simulink model "eCS_Algo_Simulation_2015b"  (R2015b)
settings: Solver=ode1  StartTime=0.0  StopTime=3  FixedStep=1/80000  RelTol=1e-3
PreLoadFcn:
  | if exist('tl_preloadfcn','file'), tl_preloadfcn(gcs,402); end
PostLoadFcn:
  | , if any(exist('dsrtsu_mdlpostloadfcn', 'file') == [2, 3, 6]), try dsrtsu_mdlpostloadfcn('Execute', bdroot); catch fprintf('Error in PostLoadFcn (dsrtsu_mdlpostloadfcn) for model "%s":\n %s\n', bdroot, lasterr); end, end,
  | if exist('tl_postloadfcn','file'), tl_postloadfcn(gcs,402); end
InitFcn:
  | Omegan=1.3024e+03;
  | xi=0.9; %0.48
  | K=0.1931;
  | K1=0.0198;
  | TauLocked=0.00255;
  | TauUnLocked=0.0042;
  | Kp=1/(2*K1);
  | Ki=Kp/((TauLocked+TauUnLocked)/2);
  | if exist('tlds_init','file'), tlds_init(gcs); end
StartFcn:
  | if exist('tlds_start','file'), tlds_start(gcs); end
StopFcn:
  | if exist('tlds_stop','file'), tlds_stop(gcs); end
model workspace (MAT data in the model file):
  au8PrevExecProfile = [0 0 0 0 0 0]
values from neighbouring files (symbols this model uses):
  AccSensor = 5    [Parameter_eCS_Algo.m]
  AlgoType = 0    [Parameter_eCS_Algo.m]
  Cxy = 1*0.017    (= 0.017)    [Acc_Init_SelV1.m]
  Cxz = 1*0.017    (= 0.017)    [Acc_Init_SelV1.m]
  Cyx = 1*0.017    (= 0.017)    [Acc_Init_SelV1.m]
  Cyz = 1*0.017    (= 0.017)    [Acc_Init_SelV1.m]
  Czx = 1*0.017    (= 0.017)    [Acc_Init_SelV1.m]
  Czy = 1*0.017    (= 0.017)    [Acc_Init_SelV1.m]
  Forced_Oscillation = 0    [Parameter_eCS_Algo.m]    (also in run_Rotation_sim.m = run)
  FreqTemperature = 10    [Acc_Init_SelV1.m]
  MaxSensorOffset = 0.3    [Acc_Init_SelV1.m]
  Mean_x_noise = 4e-3    (= 0.004)    [Acc_Init_SelV1.m]
  Mean_y_noise = 4e-3    (= 0.004)    [Acc_Init_SelV1.m]
  Mean_z_noise = 4e-3    (= 0.004)    [Acc_Init_SelV1.m]
  ODR = 8000    [Acc_Init_SelV1.m]
  offsetcorrection_on_off = 0    [Parameter_eCS_Algo.m]
  phi_pulse_rotation = 0    [Parameter_eCS_Algo.m]    (also in run_Rotation_sim.m = angle)
  pulsetype = 2    [Parameter_eCS_Algo.m]    (also in run_simulation.m = j; run_simulation_ActiveX.m = j)
  Range = 4    [Acc_Init_SelV1.m]
  sensitivity_optimisation = 0    [Parameter_eCS_Algo.m]
  TempBias = 0    [Acc_Init_SelV1.m]
  TemperatureAmp = 0    [Acc_Init_SelV1.m]
  Var_x_noise = 1.84e-9    (= 1.84e-09)    [Acc_Init_SelV1.m]
  Var_y_noise = 2.025e-09    [Acc_Init_SelV1.m]
  Var_z_noise = 1.374e-09    [Acc_Init_SelV1.m]
  w_x = 2*pi*F_x    (= 376.991118431)    [Acc_Init_SelV1.m]
  w_y = 2*pi*F_y    (= 376.991118431)    [Acc_Init_SelV1.m]
  w_z = 2*pi*F_z    (= 376.991118431)    [Acc_Init_SelV1.m]
  x_max_temp_drift = 0.061    [Acc_Init_SelV1.m]
  x_offset_enable = 0    [Acc_Init_SelV1.m]
  x_run_to_run_drift = 0.0    (= 0)    [Acc_Init_SelV1.m]
  x_temp_co_drift = 0.000    (= 0)    [Acc_Init_SelV1.m]
  Xi_x = 0.7    [Acc_Init_SelV1.m]
  Xi_y = 0.7    [Acc_Init_SelV1.m]
  Xi_z = 0.7    [Acc_Init_SelV1.m]
  y_max_temp_drift = 0.061    [Acc_Init_SelV1.m]
  y_offset_enable = 0    [Acc_Init_SelV1.m]
  y_run_to_run_drift = 0.0    (= 0)    [Acc_Init_SelV1.m]
  y_temp_co_drift = 0.000    (= 0)    [Acc_Init_SelV1.m]
  z_max_temp_drift = 0.13    [Acc_Init_SelV1.m]
  z_offset_enable = 0    [Acc_Init_SelV1.m]
  z_run_to_run_drift = 0.0    (= 0)    [Acc_Init_SelV1.m]
  z_temp_co_drift = 0.000    (= 0)    [Acc_Init_SelV1.m]
undefined symbols (not defined in the file or in its folder): controller_sample_rate, ddv, DiscIntNeverNeededParam, gmw_roada_x__m_s__, gmw_roada_y__m_s__, gmw_roadtime_2kHz, KSF_50_a_x, KSF_50_a_y, KSF_50_time, KSG_30_a_x, KSG_30_a_y, KSG_30_time, Meldorf_HindenburgstraAcceleration_x__m_s_2_, Meldorf_HindenburgstraAcceleration_y__m_s_2_, Meldorf_HindenburgstraAcceleration_z__m_s_2_, Meldorf_HindenburgstraTime__s_, pulse_FF27, pulse_MPDB, pulse_ODB40, pulse_ODB64, pulse_USNCAP, pulsetime_FF27, pulsetime_MPDB, pulsetime_ODB40, pulsetime_ODB64, pulsetime_USNCAP, Rauasphalt_60_a_x, Rauasphalt_60_a_y, Rauasphalt_60_time, sigbuilder_block, VW_416_2kHza_x_2kHz, VW_416_2kHza_y_2kHz, VW_416_2kHztime_2kHz
libraries: simulink x29, tllib x23, tl_autosar_lib x15, simulink_extras x7, LIB_TF_G_111 x2, LIB_TF_G_12_StepControl x2, LIB_TF_G_112 x1, dspsigops x1
(part 4 of 13)

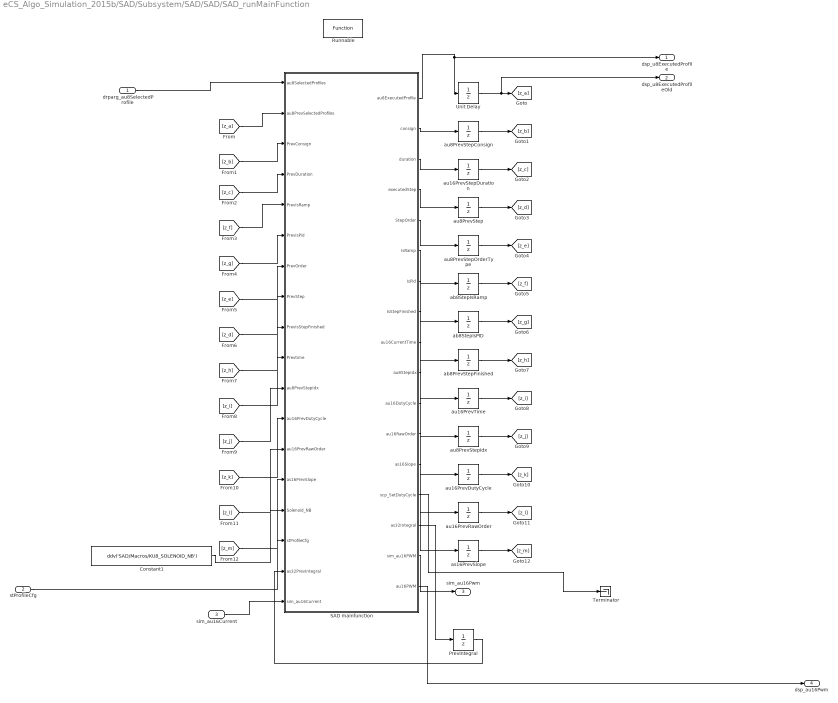
== system eCS_Algo_Simulation_2015b/SAD/Subsystem/SAD/SAD/SAD_runMainFunction ==
  drparg_au8SelectedProfile : Inport  PortDimensions=6  mask(TL_Inport){data={'logdata',{'loggingmode',1},'autosar',{'useautosarcommunication',1,'senderreceiverport','prrFsmProfile','dataelement','au8SelectedProfile'},'date',738567.35573128471}}
      settings: CopyFcn=if exist('tl_reset_reviewflag') == 2, tl_reset_reviewflag(gcbh); end  DeleteFcn=if exist('delete_tlblock','file')==2,delete_tlblock(gcbh);end  NameChangeFcn=if exist('rename_tlblock','file')==2,rename_tlblock(gcbh);end  OpenFcn=if exist('tl_open_blockdlg','file')==2,tl_open_blockdlg(gcbh);else,open_system(gcbh,'parameter');end
      mask Help: eval(['if exist(''tl_online_help'',''file'') == 2, tl_online_help(''Topic'',''TL_Inport''),else, web([''jar:file:///'',matlabroot,''/help/toolbox/simulink/help.jar!/slref/' lower(get_param(gcbh,'Blocktype')) '.html''], ''-helpbrowser''),end'])
      mask Display: plot([0.2 0.35 NaN 0.65 0.8],[0 1 NaN 0 1]);
  stProfileCfg : Inport  Port=2  mask(TL_BusInport){data={'#autoscaling',2,'#message',2,'#output',2,'#logdata',2,'logdata#1',{'loggingmode',1},'logdata#2',{'loggingmode',1},'signals',{{'stProfileCfg',{'au8FollowingProfile';'au8LastStep'}}},'autosar',{'useautosarcommunication',1,'kind',3,'interrunnablevariable','stProfileCfg'},'date',738430.41690388892}}
      settings: CopyFcn=if exist('tl_reset_reviewflag') == 2, tl_reset_reviewflag(gcbh); end  DeleteFcn=if exist('delete_tlblock','file')==2,delete_tlblock(gcbh);end  NameChangeFcn=if exist('rename_tlblock','file')==2,rename_tlblock(gcbh);end  OpenFcn=if exist('tl_open_blockdlg','file')==2,tl_open_blockdlg(gcbh);else,open_system(gcbh,'parameter');end
      mask Help: eval(['if exist(''tl_online_help'',''file'') == 2, tl_online_help(''Topic'',''TL_Inport''),else, web([''jar:file:///'',matlabroot,''/help/toolbox/simulink/help.jar!/slref/' lower(get_param(gcbh,'Blocktype')) '.html''], ''-helpbrowser''),end'])
      mask Display: plot([0.2 0.35 NaN 0.65 0.8],[0 1 NaN 0 1]);
  sim_au16Current : Inport  Port=3
  Constant1 : Constant  Value=ddv('SAD/Macros/KU8_SOLENOID_NB')  mask(TL_Constant){data={'output',{'variable','SAD/Macros/KU8_SOLENOID_NB'},'date',738430.41690414352}}
      settings: CopyFcn=if exist('tl_reset_reviewflag') == 2, tl_reset_reviewflag(gcbh); end  DeleteFcn=if exist('delete_tlblock','file')==2,delete_tlblock(gcbh);end  NameChangeFcn=if exist('rename_tlblock','file')==2,rename_tlblock(gcbh);end  OpenFcn=if exist('tl_open_blockdlg','file')==2,tl_open_blockdlg(gcbh);else,open_system(gcbh,'parameter');end
      mask Help: eval(['if exist(''tl_online_help'',''file'') == 2, tl_online_help(''Topic'',''TL_Constant''),else, web([''jar:file:///'',matlabroot,''/help/toolbox/simulink/help.jar!/slref/' lower(get_param(gcbh,'Blocktype')) '.html''], ''-helpbrowser''),end'])
      mask Display: plot([-0.1, 1.05, NaN, -0.1, 1.05],[.01, .01, NaN, .99, .99]);
  PrevIntegral : UnitDelay  InitialCondition=ddv('SAD/Vars/Steps/as32PrevIntegral')  SampleTime=-1  mask(TL_UnitDelay){data={'logdata',{'loggingmode',1},'output',{'type','Int32','scaling','scPID'},'state',{'variable','SAD/Vars/Steps/as32PrevIntegral'},'date',738433.59244626155}}
      settings: CopyFcn=if exist('tl_reset_reviewflag') == 2, tl_reset_reviewflag(gcbh); end  DeleteFcn=if exist('delete_tlblock','file')==2,delete_tlblock(gcbh);end  NameChangeFcn=if exist('rename_tlblock','file')==2,rename_tlblock(gcbh);end  OpenFcn=if exist('tl_open_blockdlg','file')==2,tl_open_blockdlg(gcbh);else,open_system(gcbh,'parameter');end
      mask Help: eval(['if exist(''tl_online_help'',''file'') == 2, tl_online_help(''Topic'',''TL_UnitDelay''),else, web([''jar:file:///'',matlabroot,''/help/toolbox/simulink/help.jar!/slref/' lower(get_param(gcbh,'Blocktype')) '.html''], ''-helpbrowser''),end'])
      mask Display: plot([-0.1, 1.05, NaN, -0.1, 1.05],[.01, .01, NaN, .99, .99]);
  Runnable : tllib/Function  data={'autosar',{'useautosarspecification',1,'softwarecomponent','AUTOLIV/SoftwareComponents/SAD/SAD','runnable','SAD_runMainFunction'},'date',738433.36681372684}  displayString=RUNNABLE
  SAD mainfunction : Subsystem  TreatAsAtomicUnit=on
  Terminator : Terminator
  Unit Delay : UnitDelay  InitialCondition=ddv('SAD/Vars/Profiles/au8PrevExecProfile')  SampleTime=-1  mask(TL_UnitDelay){data={'output',{'inheritscaling',1},'state',{'variable','SAD/Vars/Profiles/au8PrevExecProfile'},'date',738430.41691655095}}
      settings: CopyFcn=if exist('tl_reset_reviewflag') == 2, tl_reset_reviewflag(gcbh); end  DeleteFcn=if exist('delete_tlblock','file')==2,delete_tlblock(gcbh);end  NameChangeFcn=if exist('rename_tlblock','file')==2,rename_tlblock(gcbh);end  OpenFcn=if exist('tl_open_blockdlg','file')==2,tl_open_blockdlg(gcbh);else,open_system(gcbh,'parameter');end
      mask Help: eval(['if exist(''tl_online_help'',''file'') == 2, tl_online_help(''Topic'',''TL_UnitDelay''),else, web([''jar:file:///'',matlabroot,''/help/toolbox/simulink/help.jar!/slref/' lower(get_param(gcbh,'Blocktype')) '.html''], ''-helpbrowser''),end'])
      mask Display: plot([-0.1, 1.05, NaN, -0.1, 1.05],[.01, .01, NaN, .99, .99]);
  ab8PrevStepFinished : UnitDelay  InitialCondition=ddv('SAD/Vars/Steps/ab8PrevIsStepFinished')  SampleTime=-1  mask(TL_UnitDelay){data={'logdata',{'loggingmode',1},'output',{'type','Bool'},'state',{'variable','SAD/Vars/Steps/ab8PrevIsStepFinished'},'date',738430.41691681708}}
      settings: CopyFcn=if exist('tl_reset_reviewflag') == 2, tl_reset_reviewflag(gcbh); end  DeleteFcn=if exist('delete_tlblock','file')==2,delete_tlblock(gcbh);end  NameChangeFcn=if exist('rename_tlblock','file')==2,rename_tlblock(gcbh);end  OpenFcn=if exist('tl_open_blockdlg','file')==2,tl_open_blockdlg(gcbh);else,open_system(gcbh,'parameter');end
      mask Help: eval(['if exist(''tl_online_help'',''file'') == 2, tl_online_help(''Topic'',''TL_UnitDelay''),else, web([''jar:file:///'',matlabroot,''/help/toolbox/simulink/help.jar!/slref/' lower(get_param(gcbh,'Blocktype')) '.html''], ''-helpbrowser''),end'])
      mask Display: plot([-0.1, 1.05, NaN, -0.1, 1.05],[.01, .01, NaN, .99, .99]);
  ab8StepIsPID : UnitDelay  InitialCondition=ddv('SAD/Vars/Steps/astPrevSteps/Components/ab8IsPID')  SampleTime=-1  mask(TL_UnitDelay){data={'output',{'inheritscaling',1},'state',{'variable','SAD/Vars/Steps/astPrevSteps/Components/ab8IsPID'},'date',738430.41691716434}}
      settings: CopyFcn=if exist('tl_reset_reviewflag') == 2, tl_reset_reviewflag(gcbh); end  DeleteFcn=if exist('delete_tlblock','file')==2,delete_tlblock(gcbh);end  NameChangeFcn=if exist('rename_tlblock','file')==2,rename_tlblock(gcbh);end  OpenFcn=if exist('tl_open_blockdlg','file')==2,tl_open_blockdlg(gcbh);else,open_system(gcbh,'parameter');end
      mask Help: eval(['if exist(''tl_online_help'',''file'') == 2, tl_online_help(''Topic'',''TL_UnitDelay''),else, web([''jar:file:///'',matlabroot,''/help/toolbox/simulink/help.jar!/slref/' lower(get_param(gcbh,'Blocktype')) '.html''], ''-helpbrowser''),end'])
      mask Display: plot([-0.1, 1.05, NaN, -0.1, 1.05],[.01, .01, NaN, .99, .99]);
  ab8StepIsRamp : UnitDelay  InitialCondition=ddv('SAD/Vars/Steps/astPrevSteps/Components/ab8IsRamp')  SampleTime=-1  mask(TL_UnitDelay){data={'logdata',{'loggingmode',1},'output',{'inheritscaling',1},'state',{'variable','SAD/Vars/Steps/astPrevSteps/Components/ab8IsRamp'},'date',738430.41691743059}}
      settings: CopyFcn=if exist('tl_reset_reviewflag') == 2, tl_reset_reviewflag(gcbh); end  DeleteFcn=if exist('delete_tlblock','file')==2,delete_tlblock(gcbh);end  NameChangeFcn=if exist('rename_tlblock','file')==2,rename_tlblock(gcbh);end  OpenFcn=if exist('tl_open_blockdlg','file')==2,tl_open_blockdlg(gcbh);else,open_system(gcbh,'parameter');end
      mask Help: eval(['if exist(''tl_online_help'',''file'') == 2, tl_online_help(''Topic'',''TL_UnitDelay''),else, web([''jar:file:///'',matlabroot,''/help/toolbox/simulink/help.jar!/slref/' lower(get_param(gcbh,'Blocktype')) '.html''], ''-helpbrowser''),end'])
      mask Display: plot([-0.1, 1.05, NaN, -0.1, 1.05],[.01, .01, NaN, .99, .99]);
  as16PrevSlope : UnitDelay  InitialCondition=ddv('SAD/Vars/Steps/as16PrevSlope')  SampleTime=-1  mask(TL_UnitDelay){data={'output',{'inheritscaling',1},'state',{'variable','SAD/Vars/Steps/as16PrevSlope'},'date',738430.41691781254}}
      settings: CopyFcn=if exist('tl_reset_reviewflag') == 2, tl_reset_reviewflag(gcbh); end  DeleteFcn=if exist('delete_tlblock','file')==2,delete_tlblock(gcbh);end  NameChangeFcn=if exist('rename_tlblock','file')==2,rename_tlblock(gcbh);end  OpenFcn=if exist('tl_open_blockdlg','file')==2,tl_open_blockdlg(gcbh);else,open_system(gcbh,'parameter');end
      mask Help: eval(['if exist(''tl_online_help'',''file'') == 2, tl_online_help(''Topic'',''TL_UnitDelay''),else, web([''jar:file:///'',matlabroot,''/help/toolbox/simulink/help.jar!/slref/' lower(get_param(gcbh,'Blocktype')) '.html''], ''-helpbrowser''),end'])
      mask Display: plot([-0.1, 1.05, NaN, -0.1, 1.05],[.01, .01, NaN, .99, .99]);
  au16PrevDutyCycle : UnitDelay  InitialCondition=ddv('SAD/Vars/Steps/au16PrevDutyCycle')  SampleTime=-1  mask(TL_UnitDelay){data={'output',{'type','UInt16'},'state',{'variable','SAD/Vars/Steps/au16PrevDutyCycle'},'date',738566.69629486115}}
      settings: CopyFcn=if exist('tl_reset_reviewflag') == 2, tl_reset_reviewflag(gcbh); end  DeleteFcn=if exist('delete_tlblock','file')==2,delete_tlblock(gcbh);end  NameChangeFcn=if exist('rename_tlblock','file')==2,rename_tlblock(gcbh);end  OpenFcn=if exist('tl_open_blockdlg','file')==2,tl_open_blockdlg(gcbh);else,open_system(gcbh,'parameter');end
      mask Help: eval(['if exist(''tl_online_help'',''file'') == 2, tl_online_help(''Topic'',''TL_UnitDelay''),else, web([''jar:file:///'',matlabroot,''/help/toolbox/simulink/help.jar!/slref/' lower(get_param(gcbh,'Blocktype')) '.html''], ''-helpbrowser''),end'])
      mask Display: plot([-0.1, 1.05, NaN, -0.1, 1.05],[.01, .01, NaN, .99, .99]);
  au16PrevRawOrder : UnitDelay  InitialCondition=ddv('SAD/Vars/Steps/au16PrevRawOrder')  SampleTime=-1  mask(TL_UnitDelay){data={'output',{'inheritscaling',1},'state',{'variable','SAD/Vars/Steps/au16PrevRawOrder'},'date',738430.41691839125}}
      settings: CopyFcn=if exist('tl_reset_reviewflag') == 2, tl_reset_reviewflag(gcbh); end  DeleteFcn=if exist('delete_tlblock','file')==2,delete_tlblock(gcbh);end  NameChangeFcn=if exist('rename_tlblock','file')==2,rename_tlblock(gcbh);end  OpenFcn=if exist('tl_open_blockdlg','file')==2,tl_open_blockdlg(gcbh);else,open_system(gcbh,'parameter');end
      mask Help: eval(['if exist(''tl_online_help'',''file'') == 2, tl_online_help(''Topic'',''TL_UnitDelay''),else, web([''jar:file:///'',matlabroot,''/help/toolbox/simulink/help.jar!/slref/' lower(get_param(gcbh,'Blocktype')) '.html''], ''-helpbrowser''),end'])
      mask Display: plot([-0.1, 1.05, NaN, -0.1, 1.05],[.01, .01, NaN, .99, .99]);
  au16PrevStepDuration : UnitDelay  InitialCondition=ddv('SAD/Vars/Steps/astPrevSteps/Components/au16Duration')  SampleTime=-1  mask(TL_UnitDelay){data={'logdata',{'loggingmode',1},'output',{'inheritscaling',1},'state',{'variable','SAD/Vars/Steps/astPrevSteps/Components/au16Duration'},'date',738430.41691861115}}
      settings: CopyFcn=if exist('tl_reset_reviewflag') == 2, tl_reset_reviewflag(gcbh); end  DeleteFcn=if exist('delete_tlblock','file')==2,delete_tlblock(gcbh);end  NameChangeFcn=if exist('rename_tlblock','file')==2,rename_tlblock(gcbh);end  OpenFcn=if exist('tl_open_blockdlg','file')==2,tl_open_blockdlg(gcbh);else,open_system(gcbh,'parameter');end
      mask Help: eval(['if exist(''tl_online_help'',''file'') == 2, tl_online_help(''Topic'',''TL_UnitDelay''),else, web([''jar:file:///'',matlabroot,''/help/toolbox/simulink/help.jar!/slref/' lower(get_param(gcbh,'Blocktype')) '.html''], ''-helpbrowser''),end'])
      mask Display: plot([-0.1, 1.05, NaN, -0.1, 1.05],[.01, .01, NaN, .99, .99]);
  au16PrevTime : UnitDelay  InitialCondition=ddv('SAD/Vars/Steps/au16PrevTime')  SampleTime=-1  mask(TL_UnitDelay){data={'logdata',{'loggingmode',1},'output',{'inheritscaling',1},'state',{'variable','SAD/Vars/Steps/au16PrevTime'},'date',738430.41691896995}}
      settings: CopyFcn=if exist('tl_reset_reviewflag') == 2, tl_reset_reviewflag(gcbh); end  DeleteFcn=if exist('delete_tlblock','file')==2,delete_tlblock(gcbh);end  NameChangeFcn=if exist('rename_tlblock','file')==2,rename_tlblock(gcbh);end  OpenFcn=if exist('tl_open_blockdlg','file')==2,tl_open_blockdlg(gcbh);else,open_system(gcbh,'parameter');end
      mask Help: eval(['if exist(''tl_online_help'',''file'') == 2, tl_online_help(''Topic'',''TL_UnitDelay''),else, web([''jar:file:///'',matlabroot,''/help/toolbox/simulink/help.jar!/slref/' lower(get_param(gcbh,'Blocktype')) '.html''], ''-helpbrowser''),end'])
      mask Display: plot([-0.1, 1.05, NaN, -0.1, 1.05],[.01, .01, NaN, .99, .99]);
  au8PrevStep : UnitDelay  InitialCondition=ddv('SAD/Vars/Steps/au8PrevExecStep')  SampleTime=-1  mask(TL_UnitDelay){data={'output',{'inheritscaling',1},'state',{'variable','SAD/Vars/Steps/au8PrevExecStep'},'date',738430.41691923607}}
      settings: CopyFcn=if exist('tl_reset_reviewflag') == 2, tl_reset_reviewflag(gcbh); end  DeleteFcn=if exist('delete_tlblock','file')==2,delete_tlblock(gcbh);end  NameChangeFcn=if exist('rename_tlblock','file')==2,rename_tlblock(gcbh);end  OpenFcn=if exist('tl_open_blockdlg','file')==2,tl_open_blockdlg(gcbh);else,open_system(gcbh,'parameter');end
      mask Help: eval(['if exist(''tl_online_help'',''file'') == 2, tl_online_help(''Topic'',''TL_UnitDelay''),else, web([''jar:file:///'',matlabroot,''/help/toolbox/simulink/help.jar!/slref/' lower(get_param(gcbh,'Blocktype')) '.html''], ''-helpbrowser''),end'])
      mask Display: plot([-0.1, 1.05, NaN, -0.1, 1.05],[.01, .01, NaN, .99, .99]);
  au8PrevStepConsign : UnitDelay  InitialCondition=ddv('SAD/Vars/Steps/astPrevSteps/Components/au8Consign')  SampleTime=-1  mask(TL_UnitDelay){data={'output',{'inheritscaling',1},'state',{'variable','SAD/Vars/Steps/astPrevSteps/Components/au8Consign'},'date',738430.41691947915}}
      settings: CopyFcn=if exist('tl_reset_reviewflag') == 2, tl_reset_reviewflag(gcbh); end  DeleteFcn=if exist('delete_tlblock','file')==2,delete_tlblock(gcbh);end  NameChangeFcn=if exist('rename_tlblock','file')==2,rename_tlblock(gcbh);end  OpenFcn=if exist('tl_open_blockdlg','file')==2,tl_open_blockdlg(gcbh);else,open_system(gcbh,'parameter');end
      mask Help: eval(['if exist(''tl_online_help'',''file'') == 2, tl_online_help(''Topic'',''TL_UnitDelay''),else, web([''jar:file:///'',matlabroot,''/help/toolbox/simulink/help.jar!/slref/' lower(get_param(gcbh,'Blocktype')) '.html''], ''-helpbrowser''),end'])
      mask Display: plot([-0.1, 1.05, NaN, -0.1, 1.05],[.01, .01, NaN, .99, .99]);
  au8PrevStepIdx : UnitDelay  InitialCondition=ddv('SAD/Vars/Steps/au8PrevStepIdx')  SampleTime=-1  mask(TL_UnitDelay){data={'logdata',{'loggingmode',1},'output',{'inheritscaling',1},'state',{'variable','SAD/Vars/Steps/au8PrevStepIdx'},'date',738430.41691981477}}
      settings: CopyFcn=if exist('tl_reset_reviewflag') == 2, tl_reset_reviewflag(gcbh); end  DeleteFcn=if exist('delete_tlblock','file')==2,delete_tlblock(gcbh);end  NameChangeFcn=if exist('rename_tlblock','file')==2,rename_tlblock(gcbh);end  OpenFcn=if exist('tl_open_blockdlg','file')==2,tl_open_blockdlg(gcbh);else,open_system(gcbh,'parameter');end
      mask Help: eval(['if exist(''tl_online_help'',''file'') == 2, tl_online_help(''Topic'',''TL_UnitDelay''),else, web([''jar:file:///'',matlabroot,''/help/toolbox/simulink/help.jar!/slref/' lower(get_param(gcbh,'Blocktype')) '.html''], ''-helpbrowser''),end'])
      mask Display: plot([-0.1, 1.05, NaN, -0.1, 1.05],[.01, .01, NaN, .99, .99]);
  au8PrevStepOrderType : UnitDelay  InitialCondition=ddv('SAD/Vars/Steps/astPrevSteps/Components/au8OrderType')  SampleTime=-1  mask(TL_UnitDelay){data={'output',{'inheritscaling',1},'state',{'variable','SAD/Vars/Steps/astPrevSteps/Components/au8OrderType'},'date',738430.41692012735}}
      settings: CopyFcn=if exist('tl_reset_reviewflag') == 2, tl_reset_reviewflag(gcbh); end  DeleteFcn=if exist('delete_tlblock','file')==2,delete_tlblock(gcbh);end  NameChangeFcn=if exist('rename_tlblock','file')==2,rename_tlblock(gcbh);end  OpenFcn=if exist('tl_open_blockdlg','file')==2,tl_open_blockdlg(gcbh);else,open_system(gcbh,'parameter');end
      mask Help: eval(['if exist(''tl_online_help'',''file'') == 2, tl_online_help(''Topic'',''TL_UnitDelay''),else, web([''jar:file:///'',matlabroot,''/help/toolbox/simulink/help.jar!/slref/' lower(get_param(gcbh,'Blocktype')) '.html''], ''-helpbrowser''),end'])
      mask Display: plot([-0.1, 1.05, NaN, -0.1, 1.05],[.01, .01, NaN, .99, .99]);
  dsp_u8ExecutedProfile : Outport  PortDimensions=6  mask(TL_Outport){data={'logdata',{'loggingmode',1},'autosar',{'useautosarcommunication',1,'senderreceiverport','psrExecutedProfiles','dataelement','u8ExecutedProfile'},'date',738430.41692024306}}
      settings: CopyFcn=if exist('tl_reset_reviewflag') == 2, tl_reset_reviewflag(gcbh); end  DeleteFcn=if exist('delete_tlblock','file')==2,delete_tlblock(gcbh);end  NameChangeFcn=if exist('rename_tlblock','file')==2,rename_tlblock(gcbh);end  OpenFcn=if exist('tl_open_blockdlg','file')==2,tl_open_blockdlg(gcbh);else,open_system(gcbh,'parameter');end
      mask Help: eval(['if exist(''tl_online_help'',''file'') == 2, tl_online_help(''Topic'',''TL_Outport''),else, web([''jar:file:///'',matlabroot,''/help/toolbox/simulink/help.jar!/slref/' lower(get_param(gcbh,'Blocktype')) '.html''], ''-helpbrowser''),end'])
      mask Display: plot([0.2 0.35 NaN 0.65 0.8],[0 1 NaN 0 1]);
  dsp_u8ExecutedProfileOld : Outport  Port=2  PortDimensions=6  mask(TL_Outport){data={'autosar',{'useautosarcommunication',1,'senderreceiverport','psrExecutedProfiles','dataelement','u8ExecutedProfileOld'},'date',738430.4169204745}}
      settings: CopyFcn=if exist('tl_reset_reviewflag') == 2, tl_reset_reviewflag(gcbh); end  DeleteFcn=if exist('delete_tlblock','file')==2,delete_tlblock(gcbh);end  NameChangeFcn=if exist('rename_tlblock','file')==2,rename_tlblock(gcbh);end  OpenFcn=if exist('tl_open_blockdlg','file')==2,tl_open_blockdlg(gcbh);else,open_system(gcbh,'parameter');end
      mask Help: eval(['if exist(''tl_online_help'',''file'') == 2, tl_online_help(''Topic'',''TL_Outport''),else, web([''jar:file:///'',matlabroot,''/help/toolbox/simulink/help.jar!/slref/' lower(get_param(gcbh,'Blocktype')) '.html''], ''-helpbrowser''),end'])
      mask Display: plot([0.2 0.35 NaN 0.65 0.8],[0 1 NaN 0 1]);
  sim_au16Pwm : Outport  Port=3
  dsp_au16Pwm : Outport  Port=4  PortDimensions=6  mask(TL_Outport){data={'logdata',{'loggingmode',1},'autosar',{'useautosarcommunication',1,'senderreceiverport','pseSolenoidPWM','dataelement','au16Pwm'},'date',738496.37130460644}}
      settings: CopyFcn=if exist('tl_reset_reviewflag') == 2, tl_reset_reviewflag(gcbh); end  DeleteFcn=if exist('delete_tlblock','file')==2,delete_tlblock(gcbh);end  NameChangeFcn=if exist('rename_tlblock','file')==2,rename_tlblock(gcbh);end  OpenFcn=if exist('tl_open_blockdlg','file')==2,tl_open_blockdlg(gcbh);else,open_system(gcbh,'parameter');end
      mask Help: eval(['if exist(''tl_online_help'',''file'') == 2, tl_online_help(''Topic'',''TL_Outport''),else, web([''jar:file:///'',matlabroot,''/help/toolbox/simulink/help.jar!/slref/' lower(get_param(gcbh,'Blocktype')) '.html''], ''-helpbrowser''),end'])
      mask Display: plot([0.2 0.35 NaN 0.65 0.8],[0 1 NaN 0 1]);
  wires:
  SAD mainfunction/1(au8ExecutedProfile) -> Unit Delay/1, dsp_u8ExecutedProfile/1
  Unit Delay/1 -> dsp_u8ExecutedProfileOld/1, [z_a]
  drparg_au8SelectedProfile/1 -> SAD mainfunction/1(au8SelectedProfiles)
  SAD mainfunction/2(consign) -> au8PrevStepConsign/1
  SAD mainfunction/3(duration) -> au16PrevStepDuration/1
  SAD mainfunction/8(IsStepFinished) -> ab8PrevStepFinished/1
  SAD mainfunction/7(IsPid) -> ab8StepIsPID/1
  SAD mainfunction/6(IsRamp) -> ab8StepIsRamp/1
  SAD mainfunction/5(StepOrder) -> au8PrevStepOrderType/1
  SAD mainfunction/4(executedStep) -> au8PrevStep/1
  [z_a] -> SAD mainfunction/2(au8PrevSelectedProfiles)
  au8PrevStepConsign/1 -> [z_b]
  au16PrevStepDuration/1 -> [z_c]
  au8PrevStep/1 -> [z_d]
  au8PrevStepOrderType/1 -> [z_e]
  ab8StepIsRamp/1 -> [z_f]
  ab8StepIsPID/1 -> [z_g]
  ab8PrevStepFinished/1 -> [z_h]
  [z_b] -> SAD mainfunction/3(PrevConsign)
  [z_c] -> SAD mainfunction/4(PrevDuration)
  [z_f] -> SAD mainfunction/5(PrevIsRamp)
  [z_g] -> SAD mainfunction/6(PrevIsPid)
  [z_e] -> SAD mainfunction/7(PrevOrder)
  [z_d] -> SAD mainfunction/8(PrevStep)
  [z_h] -> SAD mainfunction/9(PrevIsStepFinished)
  au16PrevTime/1 -> [z_i]
  SAD mainfunction/9(au16CurrentTime) -> au16PrevTime/1
  [z_i] -> SAD mainfunction/10(Prevtime)
  SAD mainfunction/10(au8StepIdx) -> au8PrevStepIdx/1
  au8PrevStepIdx/1 -> [z_j]
  [z_j] -> SAD mainfunction/11(au8PrevStepIdx)
  [z_k] -> SAD mainfunction/12(au16PrevDutyCycle)
  SAD mainfunction/11(au16DutyCycle) -> au16PrevDutyCycle/1
  au16PrevDutyCycle/1 -> [z_k]
  SAD mainfunction/12(au16RawOrder) -> au16PrevRawOrder/1
  SAD mainfunction/13(as16Slope) -> as16PrevSlope/1
  au16PrevRawOrder/1 -> [z_l]
  as16PrevSlope/1 -> [z_m]
  [z_l] -> SAD mainfunction/13(au16PrevRawOrder)
  [z_m] -> SAD mainfunction/14(as16PrevSlope)
  Constant1/1 -> SAD mainfunction/15(Solenoid_NB)
  stProfileCfg/1 -> SAD mainfunction/16(stProfileCfg)
  SAD mainfunction/14(scp_SetDutyCycle) -> Terminator/1
  SAD mainfunction/15(as32Integral) -> PrevIntegral/1
  PrevIntegral/1 -> SAD mainfunction/17(as32PrevIntegral)
  SAD mainfunction/16(sim_au16PWM) -> sim_au16Pwm/1
  sim_au16Current/1 -> SAD mainfunction/18(sim_au16Current)
  SAD mainfunction/17(au16PWM) -> dsp_au16Pwm/1

== system eCS_Algo_Simulation_2015b/eCS/Subsystem/eCS/eCS/eCS_runMainFunction ==
  drparg_stAccelMtrPerSecSqd : Inport  mask(TL_BusInport){data={'#autoscaling',3,'#message',3,'#output',3,'#logdata',3,'logdata#1',{'loggingmode',1},'logdata#2',{'loggingmode',1},'logdata#3',{'loggingmode',1},'signals',{{'stAccelMtrPerSecSqd',{'s16Ax';'s16Ay';'s16Az'}}},'autosar',{'useautosarcommunication',1,'senderreceiverport','prrAccelMtrPerSecSqd','dataelement','stAccelMtrPerSecSqd'},'date',738573.7191865046}}
      settings: CopyFcn=if exist('tl_reset_reviewflag') == 2, tl_reset_reviewflag(gcbh); end  DeleteFcn=if exist('delete_tlblock','file')==2,delete_tlblock(gcbh);end  NameChangeFcn=if exist('rename_tlblock','file')==2,rename_tlblock(gcbh);end  OpenFcn=if exist('tl_open_blockdlg','file')==2,tl_open_blockdlg(gcbh);else,open_system(gcbh,'parameter');end
      mask Help: eval(['if exist(''tl_online_help'',''file'') == 2, tl_online_help(''Topic'',''TL_Inport''),else, web([''jar:file:///'',matlabroot,''/help/toolbox/simulink/help.jar!/slref/' lower(get_param(gcbh,'Blocktype')) '.html''], ''-helpbrowser''),end'])
      mask Display: plot([0.2 0.35 NaN 0.65 0.8],[0 1 NaN 0 1]);
  drparg_b8DiagReq : Inport  Port=2  PortDimensions=1  mask(TL_Inport){data={'autosar',{'useautosarcommunication',1,'senderreceiverport','prrEcsDiagRequest','dataelement','b8DiagReq'},'date',738573.71918724535}}
      settings: CopyFcn=if exist('tl_reset_reviewflag') == 2, tl_reset_reviewflag(gcbh); end  DeleteFcn=if exist('delete_tlblock','file')==2,delete_tlblock(gcbh);end  NameChangeFcn=if exist('rename_tlblock','file')==2,rename_tlblock(gcbh);end  OpenFcn=if exist('tl_open_blockdlg','file')==2,tl_open_blockdlg(gcbh);else,open_system(gcbh,'parameter');end
      mask Help: eval(['if exist(''tl_online_help'',''file'') == 2, tl_online_help(''Topic'',''TL_Inport''),else, web([''jar:file:///'',matlabroot,''/help/toolbox/simulink/help.jar!/slref/' lower(get_param(gcbh,'Blocktype')) '.html''], ''-helpbrowser''),end'])
      mask Display: plot([0.2 0.35 NaN 0.65 0.8],[0 1 NaN 0 1]);
  drparg_b8IsSensitivityOpt : Inport  Port=3  PortDimensions=1  mask(TL_Inport){data={'autosar',{'useautosarcommunication',1,'senderreceiverport','prrSensitivityOpt','dataelement','b8IsSensitivityOpt'},'date',738576.35882123839}}
      settings: CopyFcn=if exist('tl_reset_reviewflag') == 2, tl_reset_reviewflag(gcbh); end  DeleteFcn=if exist('delete_tlblock','file')==2,delete_tlblock(gcbh);end  NameChangeFcn=if exist('rename_tlblock','file')==2,rename_tlblock(gcbh);end  OpenFcn=if exist('tl_open_blockdlg','file')==2,tl_open_blockdlg(gcbh);else,open_system(gcbh,'parameter');end
      mask Help: eval(['if exist(''tl_online_help'',''file'') == 2, tl_online_help(''Topic'',''TL_Inport''),else, web([''jar:file:///'',matlabroot,''/help/toolbox/simulink/help.jar!/slref/' lower(get_param(gcbh,'Blocktype')) '.html''], ''-helpbrowser''),end'])
      mask Display: plot([0.2 0.35 NaN 0.65 0.8],[0 1 NaN 0 1]);
  BallAlgo : Subsystem  TreatAsAtomicUnit=on
  Bitwise Operator : tllib/Bitwise Operator  logicop=OR  UseBitMask=off  NumInputPorts=2  BitMask=bin2dec('11011001')  BitMaskRealWorld=Stored Integer  data={'date',738573.71919834486}
  Bus Selector : BusSelector  OutputSignals=s16Ax,s16Ay,s16Az
  Constant : Constant  Value=ddv('eCS_CFG/KS16_AZ_LOCK_THRS')  mask(TL_Constant){data={'output',{'variable','eCS_CFG/KS16_AZ_LOCK_THRS'},'date',738573.71919858793}}
      settings: CopyFcn=if exist('tl_reset_reviewflag') == 2, tl_reset_reviewflag(gcbh); end  DeleteFcn=if exist('delete_tlblock','file')==2,delete_tlblock(gcbh);end  NameChangeFcn=if exist('rename_tlblock','file')==2,rename_tlblock(gcbh);end  OpenFcn=if exist('tl_open_blockdlg','file')==2,tl_open_blockdlg(gcbh);else,open_system(gcbh,'parameter');end
      mask Help: eval(['if exist(''tl_online_help'',''file'') == 2, tl_online_help(''Topic'',''TL_Constant''),else, web([''jar:file:///'',matlabroot,''/help/toolbox/simulink/help.jar!/slref/' lower(get_param(gcbh,'Blocktype')) '.html''], ''-helpbrowser''),end'])
      mask Display: plot([-0.1, 1.05, NaN, -0.1, 1.05],[.01, .01, NaN, .99, .99]);
  Constant1 : Constant  Value=170  mask(TL_Constant){data={'date',738573.71919881948}}
      settings: CopyFcn=if exist('tl_reset_reviewflag') == 2, tl_reset_reviewflag(gcbh); end  DeleteFcn=if exist('delete_tlblock','file')==2,delete_tlblock(gcbh);end  NameChangeFcn=if exist('rename_tlblock','file')==2,rename_tlblock(gcbh);end  OpenFcn=if exist('tl_open_blockdlg','file')==2,tl_open_blockdlg(gcbh);else,open_system(gcbh,'parameter');end
      mask Help: eval(['if exist(''tl_online_help'',''file'') == 2, tl_online_help(''Topic'',''TL_Constant''),else, web([''jar:file:///'',matlabroot,''/help/toolbox/simulink/help.jar!/slref/' lower(get_param(gcbh,'Blocktype')) '.html''], ''-helpbrowser''),end'])
      mask Display: plot([-0.1, 1.05, NaN, -0.1, 1.05],[.01, .01, NaN, .99, .99]);
  Constant2 : Constant  Value=0  mask(TL_Constant){data={'date',738573.7191989352}}
      settings: CopyFcn=if exist('tl_reset_reviewflag') == 2, tl_reset_reviewflag(gcbh); end  DeleteFcn=if exist('delete_tlblock','file')==2,delete_tlblock(gcbh);end  NameChangeFcn=if exist('rename_tlblock','file')==2,rename_tlblock(gcbh);end  OpenFcn=if exist('tl_open_blockdlg','file')==2,tl_open_blockdlg(gcbh);else,open_system(gcbh,'parameter');end
      mask Help: eval(['if exist(''tl_online_help'',''file'') == 2, tl_online_help(''Topic'',''TL_Constant''),else, web([''jar:file:///'',matlabroot,''/help/toolbox/simulink/help.jar!/slref/' lower(get_param(gcbh,'Blocktype')) '.html''], ''-helpbrowser''),end'])
      mask Display: plot([-0.1, 1.05, NaN, -0.1, 1.05],[.01, .01, NaN, .99, .99]);
  Constant3 : Constant  mask(TL_Constant){data={'date',738573.71919905092}}
      settings: CopyFcn=if exist('tl_reset_reviewflag') == 2, tl_reset_reviewflag(gcbh); end  DeleteFcn=if exist('delete_tlblock','file')==2,delete_tlblock(gcbh);end  NameChangeFcn=if exist('rename_tlblock','file')==2,rename_tlblock(gcbh);end  OpenFcn=if exist('tl_open_blockdlg','file')==2,tl_open_blockdlg(gcbh);else,open_system(gcbh,'parameter');end
      mask Help: eval(['if exist(''tl_online_help'',''file'') == 2, tl_online_help(''Topic'',''TL_Constant''),else, web([''jar:file:///'',matlabroot,''/help/toolbox/simulink/help.jar!/slref/' lower(get_param(gcbh,'Blocktype')) '.html''], ''-helpbrowser''),end'])
      mask Display: plot([-0.1, 1.05, NaN, -0.1, 1.05],[.01, .01, NaN, .99, .99]);
  Crash Acceleration : Subsystem  TreatAsAtomicUnit=on
  Data Type Conversion : DataTypeConversion  OutDataTypeStr=boolean
  Data Type Conversion1 : DataTypeConversion  OutDataTypeStr=boolean
  Mux : Mux  Inputs=2
  Relational Operator : RelationalOperator  OutDataTypeStr=boolean  mask(TL_RelationalOperator){data={'date',738573.71920556715}}
      settings: DeleteFcn=if exist('delete_tlblock','file')==2,delete_tlblock(gcbh);end  NameChangeFcn=if exist('rename_tlblock','file')==2,rename_tlblock(gcbh);end  OpenFcn=if exist('tl_open_blockdlg','file')==2,tl_open_blockdlg(gcbh);else,open_system(gcbh,'parameter');end
      mask Help: eval(['if exist(''tl_online_help'',''file'') == 2, tl_online_help(''Topic'',''TL_RelationalOperator''),else, web([''jar:file:///'',matlabroot,''/help/toolbox/simulink/help.jar!/slref/' lower(get_param(gcbh,'Blocktype')) '.html''], ''-helpbrowser''),end'])
      mask Display: plot([-0.1, 1.05, NaN, -0.1, 1.05],[.01, .01, NaN, .99, .99]);
  Relational Operator1 : RelationalOperator  Operator===  OutDataTypeStr=boolean  mask(TL_RelationalOperator){data={'date',738573.71920568286}}
      settings: DeleteFcn=if exist('delete_tlblock','file')==2,delete_tlblock(gcbh);end  NameChangeFcn=if exist('rename_tlblock','file')==2,rename_tlblock(gcbh);end  OpenFcn=if exist('tl_open_blockdlg','file')==2,tl_open_blockdlg(gcbh);else,open_system(gcbh,'parameter');end
      mask Help: eval(['if exist(''tl_online_help'',''file'') == 2, tl_online_help(''Topic'',''TL_RelationalOperator''),else, web([''jar:file:///'',matlabroot,''/help/toolbox/simulink/help.jar!/slref/' lower(get_param(gcbh,'Blocktype')) '.html''], ''-helpbrowser''),end'])
      mask Display: plot([-0.1, 1.05, NaN, -0.1, 1.05],[.01, .01, NaN, .99, .99]);
  Runnable : tllib/Function  data={'autosar',{'useautosarspecification',1,'softwarecomponent','AUTOLIV/SoftwareComponents/eCS/eCS','runnable','eCS_runMainFunction'},'date',738492.60443505784}  displayString=RUNNABLE
  Switch : Switch  Criteria=u2 ~= 0  mask(TL_Switch){data={'output',{'type','Bool'},'date',738573.7192059143}}
      settings: CopyFcn=if exist('tl_reset_reviewflag') == 2, tl_reset_reviewflag(gcbh); end  DeleteFcn=if exist('delete_tlblock','file')==2,delete_tlblock(gcbh);end  NameChangeFcn=if exist('rename_tlblock','file')==2,rename_tlblock(gcbh);end  OpenFcn=if exist('tl_open_blockdlg','file')==2,tl_open_blockdlg(gcbh);else,open_system(gcbh,'parameter');end
      mask Help: eval(['if exist(''tl_online_help'',''file'') == 2, tl_online_help(''Topic'',''TL_Switch''),else, web([''jar:file:///'',matlabroot,''/help/toolbox/simulink/help.jar!/slref/' lower(get_param(gcbh,'Blocktype')) '.html''], ''-helpbrowser''),end'])
      mask Display: plot([-0.1, 1.05, NaN, -0.1, 1.05],[.01, .01, NaN, .99, .99]);
  eCS Latch Output : Subsystem  TreatAsAtomicUnit=on
  mToMm : Gain  Gain=ddv('MToMM')  mask(TL_Gain){data={'output',{'type','UInt16','lsb',2^-15,'unit','m'},'gain',{'variable','MToMM'},'date',738573.71921030094}}
      settings: CopyFcn=if exist('tl_reset_reviewflag') == 2, tl_reset_reviewflag(gcbh); end  DeleteFcn=if exist('delete_tlblock','file')==2,delete_tlblock(gcbh);end  NameChangeFcn=if exist('rename_tlblock','file')==2,rename_tlblock(gcbh);end  OpenFcn=if exist('tl_open_blockdlg','file')==2,tl_open_blockdlg(gcbh);else,open_system(gcbh,'parameter');end
      mask Help: eval(['if exist(''tl_online_help'',''file'') == 2, tl_online_help(''Topic'',''TL_Gain''),else, web([''jar:file:///'',matlabroot,''/help/toolbox/simulink/help.jar!/slref/' lower(get_param(gcbh,'Blocktype')) '.html''], ''-helpbrowser''),end'])
      mask Display: plot([0, .88, 0],[.05, .5, .93]);
  mergedTrigger : Logic  Operator=OR  AllPortsSameDT=off  OutDataTypeStr=boolean  mask(TL_LogicalOperator){data={'date',738573.71921041666}}
      settings: DeleteFcn=if exist('delete_tlblock','file')==2,delete_tlblock(gcbh);end  NameChangeFcn=if exist('rename_tlblock','file')==2,rename_tlblock(gcbh);end  OpenFcn=if exist('tl_open_blockdlg','file')==2,tl_open_blockdlg(gcbh);else,open_system(gcbh,'parameter');end
      mask Help: eval(['if exist(''tl_online_help'',''file'') == 2, tl_online_help(''Topic'',''TL_LogicalOperator''),else, web([''jar:file:///'',matlabroot,''/help/toolbox/simulink/help.jar!/slref/' lower(get_param(gcbh,'Blocktype')) '.html''], ''-helpbrowser''),end'])
      mask Display: plot([-0.1, 1.05, NaN, -0.1, 1.05],[.01, .01, NaN, .99, .99]);
  dsp_b8EcsFlag : Outport  PortDimensions=1  mask(TL_Outport){data={'autosar',{'useautosarcommunication',1,'senderreceiverport','psrEcsAlgoData','dataelement','b8EcsFlag'},'date',738573.71921065974}}
      settings: CopyFcn=if exist('tl_reset_reviewflag') == 2, tl_reset_reviewflag(gcbh); end  DeleteFcn=if exist('delete_tlblock','file')==2,delete_tlblock(gcbh);end  NameChangeFcn=if exist('rename_tlblock','file')==2,rename_tlblock(gcbh);end  OpenFcn=if exist('tl_open_blockdlg','file')==2,tl_open_blockdlg(gcbh);else,open_system(gcbh,'parameter');end
      mask Help: eval(['if exist(''tl_online_help'',''file'') == 2, tl_online_help(''Topic'',''TL_Outport''),else, web([''jar:file:///'',matlabroot,''/help/toolbox/simulink/help.jar!/slref/' lower(get_param(gcbh,'Blocktype')) '.html''], ''-helpbrowser''),end'])
      mask Display: plot([0.2 0.35 NaN 0.65 0.8],[0 1 NaN 0 1]);
  dsp_u16BallPosition : Outport  Port=2  PortDimensions=1  mask(TL_Outport){data={'logdata',{'loggingmode',1},'autosar',{'useautosarcommunication',1,'senderreceiverport','psrEcsAlgoData','dataelement','u16BallPosition'},'date',738573.71921085648}}
      settings: CopyFcn=if exist('tl_reset_reviewflag') == 2, tl_reset_reviewflag(gcbh); end  DeleteFcn=if exist('delete_tlblock','file')==2,delete_tlblock(gcbh);end  NameChangeFcn=if exist('rename_tlblock','file')==2,rename_tlblock(gcbh);end  OpenFcn=if exist('tl_open_blockdlg','file')==2,tl_open_blockdlg(gcbh);else,open_system(gcbh,'parameter');end
      mask Help: eval(['if exist(''tl_online_help'',''file'') == 2, tl_online_help(''Topic'',''TL_Outport''),else, web([''jar:file:///'',matlabroot,''/help/toolbox/simulink/help.jar!/slref/' lower(get_param(gcbh,'Blocktype')) '.html''], ''-helpbrowser''),end'])
      mask Display: plot([0.2 0.35 NaN 0.65 0.8],[0 1 NaN 0 1]);
  wires:
  drparg_stAccelMtrPerSecSqd/1 -> Bus Selector/1
  drparg_b8DiagReq/1 -> Relational Operator1/2
  mToMm/1 -> dsp_u16BallPosition/1
  Mux/1 -> BallAlgo/1(Pulses(x,y))
  Bus Selector/2 -> Crash Acceleration/2(Ay), Mux/2  "<s16Ay>"
  BallAlgo/1(BallPosition(m)) -> mToMm/1
  Crash Acceleration/1(b8CrashTrigger) -> mergedTrigger/2
  BallAlgo/2(BallPosTrigger) -> mergedTrigger/1
  Bus Selector/3 -> Relational Operator/1  "<s16Az>"
  Constant/1 -> Relational Operator/2
  Relational Operator/1 -> eCS Latch Output/2(b8IsAzLockReq)
  mergedTrigger/1 -> eCS Latch Output/1(b8eCSTrigger)
  Bus Selector/1 -> Crash Acceleration/1(Ax), Mux/1  "<s16Ax>"
  Relational Operator1/1 -> Switch/2
  Constant1/1 -> Relational Operator1/1
  Constant2/1 -> Switch/3
  eCS Latch Output/1(b8eCSTriggerFiltered) -> Data Type Conversion/1
  Bitwise Operator/1 -> dsp_b8EcsFlag/1
  Constant3/1 -> Switch/1
  Switch/1 -> Data Type Conversion1/1
  Data Type Conversion/1 -> Bitwise Operator/1
  Data Type Conversion1/1 -> Bitwise Operator/2
  drparg_b8IsSensitivityOpt/1 -> BallAlgo/2(b8IsSensitivityOpt)
